simulink model "lab4_2"  (R2021b)
settings: Solver=VariableStepAuto  StartTime=0.0  StopTime=20.0  RelTol=10e-10  AbsTol=10e-10
values from neighbouring files (symbols this model uses):
  d_bar = (Ra/Kt)*tau_l    (= 3)    [lab4.m]
  thetades = pi/2    (= 1.57079632679)    [lab4.m]
  TI = 1/(0.1*Output1Wcp)    [lab4.m]
  Vlim = 5    [lab4.m]
undefined symbols (not defined in the file or in its folder): Kaw
libraries: cstblocks x2
settings Model: Creator=jiayizhou  LastModifiedBy=jiayizhou

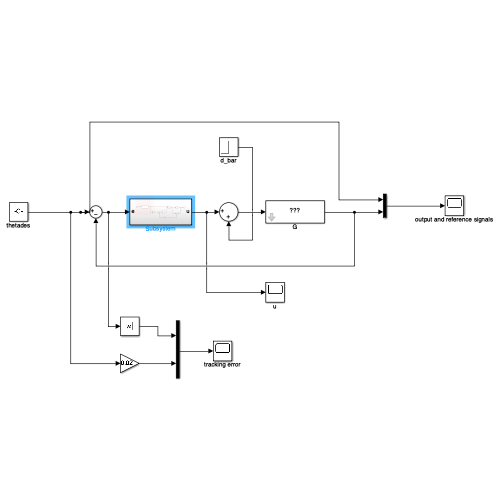
[thumbnail: Simulink's stored preview of the top-level diagram]
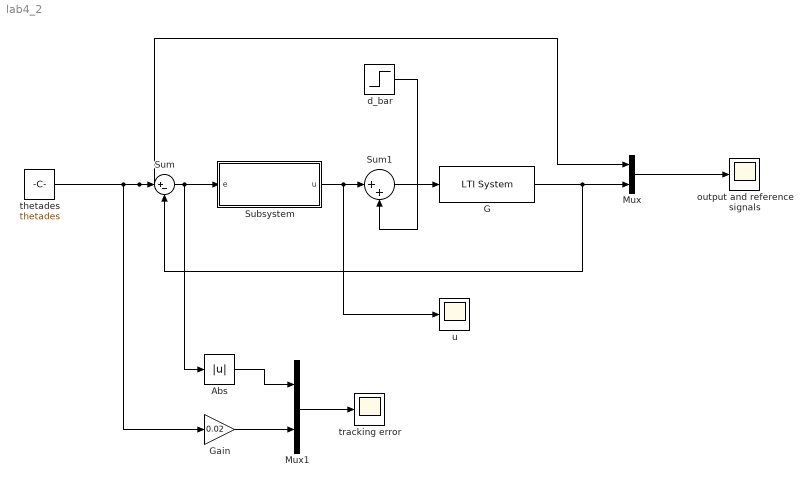
== system lab4_2 ==
  Abs : Abs
  G : cstblocks/LTI System  sys=G  IC=[]
  Gain : Gain  Gain=0.02
  Mux : Mux  Inputs=2
  Mux1 : Mux  Inputs=2
  Subsystem : Subsystem
  Sum : Sum  Inputs=|+-
  Sum1 : Sum  Inputs=|++
  d_bar : Step  Time=5  After=d_bar  SampleTime=0
  output and reference signals : Scope
  thetades : Constant  Value=thetades
  tracking error : Scope
  u : Scope
  wires:
  Mux/1 -> output and reference signals/1
  d_bar/1 -> Sum1/2
  thetades/1 -> Gain/1, Mux/1, Sum/1
  Sum/1 -> Subsystem/1(e), Abs/1
  Sum1/1 -> G/1
  Mux1/1 -> tracking error/1
  Gain/1 -> Mux1/2
  G/1 -> Mux/2, Sum/2
  Abs/1 -> Mux1/1
  Subsystem/1(u) -> u/1, Sum1/1

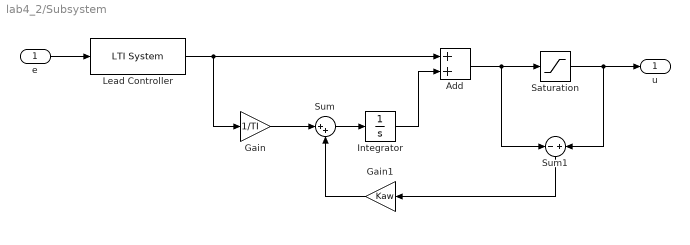
== system lab4_2/Subsystem ==
  e : Inport
  Add : Sum
  Gain : Gain  Gain=1/TI
  Gain1 : Gain  Gain=Kaw
  Integrator : Integrator
  Lead Controller : cstblocks/LTI System  sys=C1  IC=[]
  Saturation : Saturate  UpperLimit=Vlim  LowerLimit=-Vlim
  Sum : Sum  Inputs=|++
  Sum1 : Sum  Inputs=-|+
  u : Outport
  wires:
  e/1 -> Lead Controller/1
  Lead Controller/1 -> Gain/1, Add/1
  Gain/1 -> Sum/1
  Gain1/1 -> Sum/2
  Sum/1 -> Integrator/1
  Integrator/1 -> Add/2
  Add/1 -> Sum1/1, Saturation/1
  Saturation/1 -> Sum1/2, u/1
  Sum1/1 -> Gain1/1
